simulink model "powamp_dpd"  (R2022a)
settings: Solver=FixedStepAuto  StartTime=0.0  StopTime=2e-4  RelTol=1e-3
PreLoadFcn:
  | [txWaveform,BW] = helperPACharGenerateTones();
  | Tstep = 1/BW;                   %  Simulation BW BB
  | RF = 3.7e9;                       %  RF center frequency
  | IF = 500e6;                          % IF frequency
  | dataRatePA = 1/BW;  % PA characterization sample time
  | HPF_cutoff = RF - 500e6;
  | 
  | overSamplingRate = 7;
  | filterLength = 6*70;
  | lowpassfilter = firpm(filterLength, [0 8/70 10/70 1], [1 1 0 0]);
  | firInterp = dsp.FIRInterpolator(overSamplingRate, lowpassfilter);
  | txWaveformInterp = firInterp([txWaveform; zeros(filterLength/overSamplingRate/2,1)]);
  | txWaveformInterp = txWaveformInterp((filterLength/2)+1:end,1);      % Remove transients
  | 
  | dataFileName = "helperPACharSavedDataTones";
  | load(dataFileName,"results","sampleRate","overSamplingRate","testSignal","numFrames")
  | 
  | paInput = results.InputWaveform;
  | paOutput = results.OutputWaveform;
  | modType = 'memPoly';
  | memLen = 5;
  | degLen = 5;
  | halfDataPts = round(length(paInput)/2);
  | origState = warning;
  | warning('off', 'MATLAB:rankDeficientMatrix')
  | paModelMemPoly = double(helperPACharMemPolyModel('coefficientFinder', ...
  |   paInput(1:halfDataPts),paOutput(1:halfDataPts),memLen,degLen,modType));
  | warning(origState);
  | 
  | gain = results.LinearGain;
  | scaleFactor = double(max(abs(paOutput))/max(abs(txWaveformInterp))/gain);
undefined symbols (not defined in the file or in its folder): S
libraries: simrfV2elements x8, simrfV2util1 x4, commrfcorlib x2, simrfV2systems x2, simrfV2_lib x2, simrfV2junction1 x1, dspmlti4 x1, dspsrcs4 x1
Description:
  | Power Amplifier Characterization with DPD for Reduced Signal Distortion
settings Model: SimulationMode=accelerator  Creator=The MathWorks, Inc.  LastModifiedBy=Administrator
settings SolverCC: ZeroCrossAlgorithm=Adaptive  AlgebraicLoopSolver=TrustRegion
settings DataIOCC: LimitDataPoints=on  SaveFormat=Array  SaveOutput=off  SignalLogging=off  DSMLogging=off  SaveTime=off  ReturnWorkspaceOutputs=off
settings OptimizationCC: BlockReduction=off  BooleanDataType=off  LifeSpan=inf
settings DebuggingCC: SaveWithParameterizedLinksMsg=none  UnderspecifiedInitializationDetection=Classic  MergeDetectMultiDrivingBlocksExec=none  SignalResolutionControl=TryResolveAllWithWarning  UnconnectedInputMsg=warning  UnconnectedOutputMsg=warning  UnconnectedLineMsg=warning  AllowSymbolicDim=off  SFUnexpectedBacktrackingDiag=warning  SFNoUnconditionalDefaultTransitionDiag=warning  SFExecutionAtInitializationDiag=none  SFMachineParentedDataDiag=warning  ArithmeticOperatorsInVariantConditions=warning
settings HardwareCC: ProdBitPerPointer=32  ProdBitPerSizeT=32  ProdBitPerPtrDiffT=32  ProdLargestAtomicFloat=None  ProdIntDivRoundTo=Undefined  ProdEndianess=Unspecified  ProdWordSize=32  ProdHWDeviceType=32-bit Generic  TargetBitPerPointer=64  TargetBitPerSizeT=64  TargetBitPerPtrDiffT=64  TargetLongLongMode=on  TargetIntDivRoundTo=Zero  TargetEndianess=LittleEndian  TargetWordSize=64  TargetHWDeviceType=MATLAB Host  ProdEqTarget=off
settings ModelReferenceCC: PropagateSignalLabelsOutOfModel=off
settings SFSimCC: SimUseLocalCustomCode=off  CustomCodeUndefinedFunction=UseInterfaceOnly
settings RTWCC: RTWUseLocalCustomCode=off  BuildConfiguration=Faster Runs  DLArmComputeVersion=19.05
settings CodeAppCC: StateflowObjectComments=on
settings GRTTargetCC: TargetLangStandard=C89/C90 (ANSI)
settings ConfigComp: CovMetricSettings=dw  CovSaveCumulativeToWorkspaceVar=on  CovSaveSingleToWorkspaceVar=on  CovExternalEMLEnable=off
settings SimscapeCC: SimscapeNormalizeSystem=off

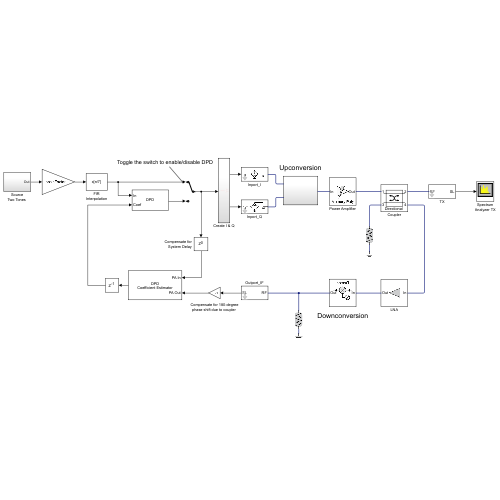
[thumbnail: Simulink's stored preview of the top-level diagram]
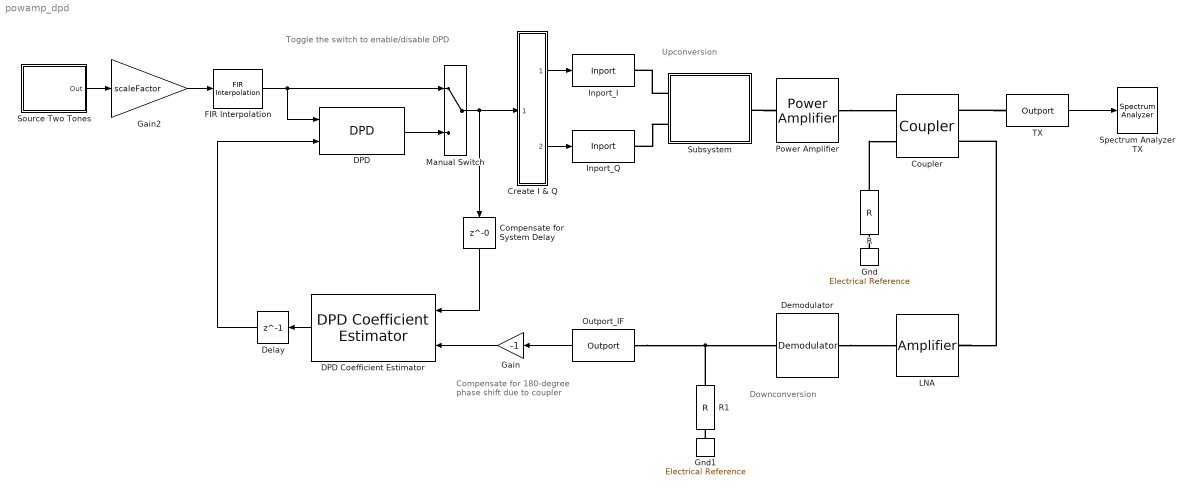
== system powamp_dpd ==
  note: Toggle the switch to enable/disable DPD
  note: Compensate for 180-degree
      | phase shift due to coupler
  note: Downconversion
  note: Upconversion
  Compensate for System Delay : Delay  DelayLength=0
  Coupler : simrfV2junction1/Coupler  classname=couplers  DataSource=Network-parameters  NumPorts=4  DeviceCirculator=Circulator clockwise  DeviceDivider=T power divider  DeviceCoupler=Directional coupler  Paramtype=S-parameters  Sparam=[0 0 1; 1 0 0; 0 1 0]  SparamFreq=1e9 Hz  SparamZ0=50  Phase12=0  Phase33=0  Alpha=0  Coupling=55  Directivity=inf  InsertionLoss=0.0001  ReturnLoss=inf  InternalGrounding=on  SparamRepresentation=Frequency domain  FitOpt=Share all poles  FitTol=-40  MaxPoles=48
      settings: SourceProductBaseCode=RB
  Create I & Q : Subsystem
  DPD : commrfcorlib/DPD  PolynomialType=Memory polynomial  CoefficientSource=Input port  Coefficients=complex([1 0 0 0 0; 0 0 0 0 0; 0 0 0 0 0])  SimulateUsing=Code generation
      settings: SourceProductBaseCode=CM
  DPD Coefficient Estimator : commrfcorlib/DPD Coefficient Estimator  DesiredAmplitudeGaindB=10*log10(gain)  PolynomialType=Memory polynomial  Degree=3  MemoryDepth=5  Algorithm=Recursive least squares  ForgettingFactorSource=Property  ForgettingFactor=0.999  InitialCoefficientEstimate=[]  SimulateUsing=Code generation
      settings: SourceProductBaseCode=CM
  Delay : Delay  DelayLength=1
  Demodulator : simrfV2systems/Demodulator  classname=rfdemod  Source_linear_gain=Available power gain  linear_gain=0 dB  Poly_Coeffs=[0 1]  LOFreq=RF-IF Hz  Zin=50  Zout=50  AddIRFilter=on  AddCSFilter=off  InternalGrounding=on  ForceNextInit=off  Source_Poly=Even and odd order  IPType=Input  IP2=inf dBm  IP3=inf dBm  P1dB=inf dBm  Psat=inf dBm  Gcomp=inf dBm  NF=1  Isolation=inf dB  AddPhaseNoise=off  PhaseNoiseOffset=[5e5 1e6 5e6]  PhaseNoiseLevel=[-108 -130 -140]  AutoImpulseLengthPN=on  ImpulseLengthPN=1e-10  ImpulseLength_unitPN=s  DesignMethodIR=Ideal  ResponseTypeIR=Highpass  ImplementationIR=LC Tee  ImplementationIdealIR=Constant per carrier  ImplementationRationalIR=Transfer function  UseFilterOrderIR=on  FilterOrderIR=3  PassFreq_lpIR=1  PassFreq_lp_unitIR=GHz  PassFreq_hpIR=HPF_cutoff  PassFreq_hp_unitIR=Hz  PassFreq_bpIR=[2 3]  PassFreq_bp_unitIR=GHz  PassFreq_bsIR=[1 4]  PassFreq_bs_unitIR=GHz  PassAttenIR=10*log10(2)  StopFreq_lpIR=2  StopFreq_lp_unitIR=GHz  StopFreq_hpIR=1  StopFreq_hp_unitIR=GHz  StopFreq_bpIR=[1.5 3.5]  StopFreq_bp_unitIR=GHz  StopFreq_bsIR=[2.1 2.9]  StopFreq_bs_unitIR=GHz  StopAttenIR=40  RsrcIR=50  RloadIR=50  AutoImpulseLengthIR=on  ImpulseLengthIR=1e-10  ImpulseLength_unitIR=s  DesignMethodCS=Ideal  ResponseTypeCS=Lowpass  ImplementationCS=LC Tee  ImplementationIdealCS=Constant per carrier  ImplementationRationalCS=Transfer function  UseFilterOrderCS=on  FilterOrderCS=3  PassFreq_lpCS=1  PassFreq_lp_unitCS=GHz  PassFreq_hpCS=2  PassFreq_hp_unitCS=GHz  PassFreq_bpCS=[2 3]  PassFreq_bp_unitCS=GHz  PassFreq_bsCS=[1 4]  PassFreq_bs_unitCS=GHz  PassAttenCS=10*log10(2)  StopFreq_lpCS=2  StopFreq_lp_unitCS=GHz  StopFreq_hpCS=1  StopFreq_hp_unitCS=GHz  StopFreq_bpCS=[1.5 3.5]  StopFreq_bp_unitCS=GHz  StopFreq_bsCS=[2.1 2.9]  StopFreq_bs_unitCS=GHz  StopAttenCS=40  RsrcCS=50  RloadCS=50  AutoImpulseLengthCS=on  ImpulseLengthCS=1e-10  ImpulseLength_unitCS=s
      settings: SourceProductBaseCode=RB
  FIR Interpolation : dspmlti4/FIR Interpolation  FilterSource=Dialog parameters  PrivateCoeffs=0  h=firpm(filterLength, [0 8/70 10/70 1], [1 1 0 0])  L=overSamplingRate  FilterObject=FINTERP  InputProcessing=Columns as channels (frame based)  framing=Allow multirate processing  outputBufInitCond=0  roundingMode=Floor  overflowMode=off  firstCoeffDataTypeStr=Inherit: Same word length as input  firstCoeffMin=[]  firstCoeffMax=[]  firstCoeffLastDataTypeStr=Inherit: Same word length as input  outputDataTypeStr=Inherit: Same as accumulator  outputMin=[]  outputMax=[]  outputLastDataTypeStr=Inherit: Same as accumulator
  Gain : Gain  Gain=-1
  Gain2 : Gain  Gain=scaleFactor
  Gnd : simrfV2_lib/Elements/Electrical Reference
      settings: SourceProductBaseCode=RB  InternalSimscapePortConfiguration="{\"Bottom\":[],\"Left\":[{\"id\":\"V\",\"label\":\"\",\"type\":\"foundation.rf.circuitenvelope\"}],\"Right\":[],\"Top\":[]}"
  Gnd1 : simrfV2_lib/Elements/Electrical Reference
      settings: SourceProductBaseCode=RB  InternalSimscapePortConfiguration="{\"Bottom\":[],\"Left\":[{\"id\":\"V\",\"label\":\"\",\"type\":\"foundation.rf.circuitenvelope\"}],\"Right\":[],\"Top\":[]}"
  Inport_I : simrfV2util1/Inport  SimulinkInputSignalType=Ideal voltage  CarrierFreq=0 Hz  ZS=0  InternalGrounding=on
      settings: SourceProductBaseCode=RB
  Inport_Q : simrfV2util1/Inport  SimulinkInputSignalType=Ideal voltage  CarrierFreq=0 Hz  ZS=0  InternalGrounding=on
      settings: SourceProductBaseCode=RB
  LNA : simrfV2elements/Amplifier  classname=amplifier  DataSource=Data file  File=unitygain.s2p  Paramtype=S-parameters  Sparam=[0 0;1 0]  SparamFreq=1e9 Hz  SparamZ0=50  Residues=0  Poles=0  DF={0 0; 1 0}  Source_linear_gain=Available power gain  linear_gain=55 dB  AmAmAmPmTable=[-25,5,-1;-10,20,-2;0,27,5;5,28,12]  Zin=50  Zout=50  Source_Poly=Odd order  Poly_Coeffs=[0 1]  IPType=Output  IP2=19.5 dBm  IP3=inf dBm  P1dB=inf dBm  Psat=inf dBm  Gcomp=inf dBm  InternalGrounding=on  SourceFreq=Extracted from data source  PlotFreq=0 Hz  PlotType=X-Y plane  YParam1=S(1,1)  YFormat1=Magnitude (decibels)  YParam2=None  YFormat2=Magnitude (decibels)  YOption=Linear  XOption=Linear  SparamRepresentation=Time domain (rationalfit)  FitTol=-40  FitOpt=Share all poles  MaxPoles=48  AutoImpulseLength=off  ImpulseLength=0 s  MagModeling=off  AddNoise=on  NoiseType=Noise figure  NoiseDist=White  NF=0.1  MinNF=0  Gopt=0  RN=0  CarrierFreq=0 Hz  NoiseAutoImpulseLength=on  NoiseImpulseLength=1e-10 s  ConstS21NL=on  OpFreq=0 Hz  SetOpFreqAsMaxS21=on
      settings: SourceProductBaseCode=RB
  Manual Switch : ManualSwitch
  Outport_IF : simrfV2util1/Outport  SensorType=Ideal voltage  OutputFormat=Complex Baseband  CarrierFreq=IF Hz  ZL=Inf  InternalGrounding=on  StepSize=-1 s  AutoStep=off
      settings: SourceProductBaseCode=RB
  Power Amplifier : simrfV2elements/Power Amplifier  classname=poweramp  ModelType=Memory polynomial  CoeffMatrix=paModelMemPoly  UnitDelay=dataRatePA/overSamplingRate  Rin=50  Rout=50  InternalGrounding=on
      settings: SourceProductBaseCode=RB
  R : simrfV2elements/R  classname=resistor  Resistance=50 Ohm  AddNoise=on
      settings: SourceProductBaseCode=RB
  R1 : simrfV2elements/R  classname=resistor  Resistance=50 Ohm  AddNoise=on
      settings: SourceProductBaseCode=RB
  "Source Two Tones " : Subsystem
  Spectrum Analyzer TX : SpectrumAnalyzer
  Subsystem : Subsystem
  TX : simrfV2util1/Outport  SensorType=Ideal voltage  OutputFormat=Complex Baseband  CarrierFreq=RF Hz  ZL=Inf  InternalGrounding=on  StepSize=-1 s  AutoStep=off
      settings: SourceProductBaseCode=RB
  wires:
  TX/1 -> Spectrum Analyzer TX/1
  Compensate for System Delay/1 -> DPD Coefficient Estimator/1
  FIR Interpolation/1 -> DPD/1, Manual Switch/1
  Create I & Q/1(Out1) -> Inport_I/1
  Outport_IF/1 -> Gain/1
  DPD/1 -> Manual Switch/2
  "Source Two Tones "/1(Out) -> Gain2/1
  DPD Coefficient Estimator/1 -> Delay/1
  Gain2/1 -> FIR Interpolation/1
  Delay/1 -> DPD/2
  Gain/1 -> DPD Coefficient Estimator/2
  Create I & Q/2(Out2) -> Inport_Q/1
  Manual Switch/1 -> Compensate for System Delay/1, Create I & Q/1(In1)
  connections:
  TX/LConn1 -- Coupler/RConn1
  Outport_IF/LConn1 -- Demodulator/RConn1 -- R1/LConn1
  LNA/LConn1 -- Coupler/RConn2
  R/LConn1 -- Coupler/LConn2
  Gnd1/LConn1 -- R1/RConn1
  Gnd/LConn1 -- R/RConn1
  Demodulator/LConn1 -- LNA/RConn1
  Subsystem/LConn2 -- Inport_Q/RConn1
  Power Amplifier/LConn1 -- Subsystem/RConn1
  Subsystem/LConn1 -- Inport_I/RConn1
  Power Amplifier/RConn1 -- Coupler/LConn1

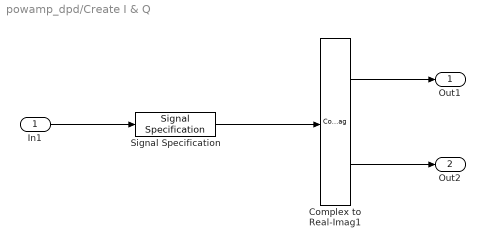
== system powamp_dpd/Create I & Q ==
  In1 : Inport
  Complex to Real-Imag1 : ComplexToRealImag
  Signal Specification : SignalSpecification  Dimensions=1
  Out1 : Outport  VectorParamsAs1DForOutWhenUnconnected=off
  Out2 : Outport  Port=2  VectorParamsAs1DForOutWhenUnconnected=off
  wires:
  Complex to Real-Imag1/1 -> Out1/1
  Complex to Real-Imag1/2 -> Out2/1
  In1/1 -> Signal Specification/1
  Signal Specification/1 -> Complex to Real-Imag1/1

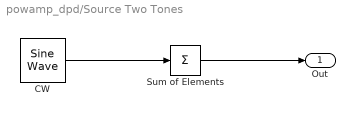
== system powamp_dpd/Source Two Tones  ==
  CW : dspsrcs4/Sine Wave  Amplitude=[1 1]  Frequency=[1.8 2.6]*1e6  Phase=0  SampleMode=Discrete  OutComplex=Complex  CompMethod=Trigonometric fcn  TableSize=Speed  SampleTime=Tstep  SamplesPerFrame=1  ResetState=Restart at time zero  OutputFrames=off  dataType=double  wordLen=16  udDataType=sfix(16)  fracBitsMode=Best precision  numFracBits=15  OutDataTypeStr=double  LastOutDataTypeStr=double
  Sum of Elements : Sum  Inputs=+  CollapseMode=Specified dimension  CollapseDim=2
  Out : Outport  VectorParamsAs1DForOutWhenUnconnected=off
  wires:
  CW/1 -> Sum of Elements/1
  Sum of Elements/1 -> Out/1

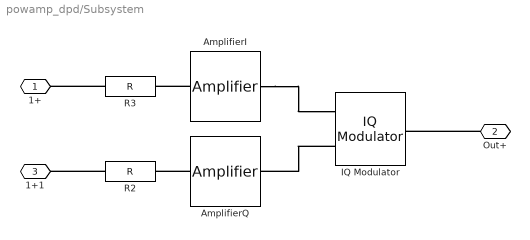
== system powamp_dpd/Subsystem ==
  AmplifierI : simrfV2elements/Amplifier  classname=amplifier  DataSource=Data file  File=unitygain.s2p  Paramtype=S-parameters  Sparam=[0 0;1 0]  SparamFreq=1e9 Hz  SparamZ0=50  Residues=0  Poles=0  DF={0 0; 1 0}  Source_linear_gain=Available power gain  linear_gain=10*log10(4) dB  AmAmAmPmTable=[-25,5,-1;-10,20,-2;0,27,5;5,28,12]  Zin=50  Zout=50  Source_Poly=Even and odd order  Poly_Coeffs=[0 1]  IPType=Input  IP2=inf dBm  IP3=inf dBm  P1dB=inf dBm  Psat=inf dBm  Gcomp=inf dBm  InternalGrounding=on  SourceFreq=Extracted from data source  PlotFreq=[1e9:1e6:3e9] Hz  PlotType=X-Y plane  YParam1=S(1,1)  YFormat1=Magnitude (decibels)  YParam2=None  YFormat2=Magnitude (decibels)  YOption=Linear  XOption=Linear  SparamRepresentation=Time domain (rationalfit)  FitTol=-40  FitOpt=Fit individually  MaxPoles=48  AutoImpulseLength=on  ImpulseLength=1e-10 s  MagModeling=off  AddNoise=on  NoiseType=Noise figure  NoiseDist=White  NF=0.2  MinNF=0  Gopt=0  RN=0  CarrierFreq=0 Hz  NoiseAutoImpulseLength=on  NoiseImpulseLength=1e-10 s  ConstS21NL=on  OpFreq=0 Hz  SetOpFreqAsMaxS21=on
      settings: SourceProductBaseCode=RB
  AmplifierQ : simrfV2elements/Amplifier  classname=amplifier  DataSource=Data file  File=unitygain.s2p  Paramtype=S-parameters  Sparam=[0 0;1 0]  SparamFreq=1e9 Hz  SparamZ0=50  Residues=0  Poles=0  DF={0 0; 1 0}  Source_linear_gain=Available power gain  linear_gain=10*log10(4) dB  AmAmAmPmTable=[-25,5,-1;-10,20,-2;0,27,5;5,28,12]  Zin=50  Zout=50  Source_Poly=Even and odd order  Poly_Coeffs=[0 1]  IPType=Input  IP2=inf dBm  IP3=inf dBm  P1dB=inf dBm  Psat=inf dBm  Gcomp=inf dBm  InternalGrounding=on  SourceFreq=Extracted from data source  PlotFreq=[1e9:1e6:3e9] Hz  PlotType=X-Y plane  YParam1=S(1,1)  YFormat1=Magnitude (decibels)  YParam2=None  YFormat2=Magnitude (decibels)  YOption=Linear  XOption=Linear  SparamRepresentation=Time domain (rationalfit)  FitTol=-40  FitOpt=Fit individually  MaxPoles=48  AutoImpulseLength=on  ImpulseLength=1e-10 s  MagModeling=off  AddNoise=on  NoiseType=Noise figure  NoiseDist=White  NF=0.2  MinNF=0  Gopt=0  RN=0  CarrierFreq=0 Hz  NoiseAutoImpulseLength=on  NoiseImpulseLength=1e-10 s  ConstS21NL=on  OpFreq=0 Hz  SetOpFreqAsMaxS21=on
      settings: SourceProductBaseCode=RB
  IQ Modulator : simrfV2systems/IQ Modulator  classname=iqmod  Source_linear_gain=Available power gain  linear_gain=10*log10(2) dB  Poly_Coeffs=[0 1]  LOFreq=RF Hz  Zin=50  Zout=50  AddIRFilters=off  AddCSFilter=on  InternalGrounding=on  ForceNextInit=off  NFloor=-inf  GainMismatch=0 dB  PhaseMismatch=0 deg  Isolation=inf dB  AddPhaseNoise=off  PhaseNoiseOffset=1e6  PhaseNoiseLevel=-140  AutoImpulseLengthPN=on  ImpulseLengthPN=1e-10  ImpulseLength_unitPN=s  Source_Poly=Even and odd order  IPType=Input  IP2=inf dBm  IP3=inf dBm  P1dB=inf dBm  Psat=inf dBm  Gcomp=inf dBm  DesignMethodIR=Ideal  ResponseTypeIR=Lowpass  ImplementationIR=LC Tee  ImplementationIdealIR=Constant per carrier  ImplementationRationalIR=Transfer function  UseFilterOrderIR=on  FilterOrderIR=3  PassFreq_lpIR=1  PassFreq_lp_unitIR=GHz  PassFreq_hpIR=2  PassFreq_hp_unitIR=GHz  PassFreq_bpIR=[2 3]  PassFreq_bp_unitIR=GHz  PassFreq_bsIR=[1 4]  PassFreq_bs_unitIR=GHz  PassAttenIR=10*log10(2)  StopFreq_lpIR=2  StopFreq_lp_unitIR=GHz  StopFreq_hpIR=1  StopFreq_hp_unitIR=GHz  StopFreq_bpIR=[1.5 3.5]  StopFreq_bp_unitIR=GHz  StopFreq_bsIR=[2.1 2.9]  StopFreq_bs_unitIR=GHz  StopAttenIR=40  RsrcIR=50  RloadIR=50  AutoImpulseLengthIR=on  ImpulseLengthIR=1e-10  ImpulseLength_unitIR=s  DesignMethodCS=Ideal  ResponseTypeCS=Highpass  ImplementationCS=LC Tee  ImplementationIdealCS=Constant per carrier  ImplementationRationalCS=Transfer function  UseFilterOrderCS=on  FilterOrderCS=3  PassFreq_lpCS=1  PassFreq_lp_unitCS=GHz  PassFreq_hpCS=HPF_cutoff  PassFreq_hp_unitCS=Hz  PassFreq_bpCS=[2 3]  PassFreq_bp_unitCS=GHz  PassFreq_bsCS=[1 4]  PassFreq_bs_unitCS=GHz  PassAttenCS=10*log10(2)  StopFreq_lpCS=2  StopFreq_lp_unitCS=GHz  StopFreq_hpCS=1  StopFreq_hp_unitCS=GHz  StopFreq_bpCS=[1.5 3.5]  StopFreq_bp_unitCS=GHz  StopFreq_bsCS=[2.1 2.9]  StopFreq_bs_unitCS=GHz  StopAttenCS=40  RsrcCS=50  RloadCS=50  AutoImpulseLengthCS=on  ImpulseLengthCS=1e-10  ImpulseLength_unitCS=s
      settings: SourceProductBaseCode=RB
  R2 : simrfV2elements/R  classname=resistor  Resistance=50 Ohm  AddNoise=on
      settings: SourceProductBaseCode=RB
  R3 : simrfV2elements/R  classname=resistor  Resistance=50 Ohm  AddNoise=on
      settings: SourceProductBaseCode=RB
  1+ : PMIOPort  Side=Left
  Out+ : PMIOPort  Port=2  Side=Right
  1+1 : PMIOPort  Port=3  Side=Left
  connections:
  Out+/RConn1 -- IQ Modulator/RConn1
  IQ Modulator/LConn2 -- AmplifierQ/RConn1
  AmplifierI/LConn1 -- R3/RConn1
  AmplifierI/RConn1 -- IQ Modulator/LConn1
  R3/LConn1 -- 1+/RConn1
  AmplifierQ/LConn1 -- R2/RConn1
  R2/LConn1 -- 1+1/RConn1
